simulink model "function_model"  (R2018a)
settings: Solver=VariableStepAuto  StartTime=0.0  StopTime=10.0  RelTol=1e-3
settings Model: Creator=FPR9FE  LastModifiedBy=FPR9FE

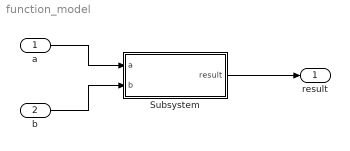
== system function_model ==
  a : Inport
  b : Inport  Port=2
  Subsystem : Subsystem
  result : Outport
  wires:
  Subsystem/1(result) -> result/1
  a/1 -> Subsystem/1(a)
  b/1 -> Subsystem/2(b)

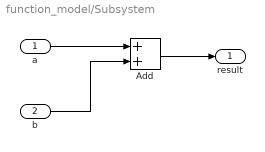
== system function_model/Subsystem ==
  a : Inport
  b : Inport  Port=2
  Add : Sum
  result : Outport
  wires:
  a/1 -> Add/1
  b/1 -> Add/2
  Add/1 -> result/1
